simulink model "F16ASYM_Controlled"  (R2015a)
settings: Solver=ode3  SolverMode=SingleTasking  StartTime=0.0  StopTime=inf  FixedStep=T_sim  RelTol=1e-3
InitFcn:
  | load('NN_c_weights_Last_stable.mat')
StopFcn:
  | Final_results
values from neighbouring files (symbols this model uses):
  a1 = fitresult.p1    [Stall_protection.m]
  alpha_map_eval = ones(size(M_eval))*NaN    [Auto_trim_aid.m]    (also in Autotrim_maps.mat = [nan nan 0.277598136245 0.119432432992 0.0579479097061 0.027)
  beta_map_eval = ones(size(M_eval))*NaN    [Auto_trim_aid.m]    (also in Autotrim_maps.mat = [nan nan -0.00151549403324 0.00117807579006 -0.0052086799721)
  C_L_0 = fitresult.p2    [Stall_protection.m]
  G_eval = NaN*ones(size(M_sq,2),size(H_sq,2))    [Stall_protection.m]
  H_sq = unique(sort(H_sq))    [Stall_protection.m]
  H_sq_autotrim = min( F_envelope.H_1g):2000:max(F_envelope.H_1g)    [Auto_trim_aid.m]    (also in Autotrim_maps.mat = [0 2000 4000 6000 8000 10000 12000 14000 16000 18000])
  K_b_q_extrap_ACC = K_b_q_extrap    [RUN_ME.m]
  K_b_q_extrap_AoA = K_b_q_extrap    [RUN_ME.m]
  M_sq = unique(sort(M_sq))    [Stall_protection.m]
  M_sq_autotrim = 0:0.1:max(F_envelope.M_1g)    [Auto_trim_aid.m]    (also in Autotrim_maps.mat = [0 0.1 0.2 0.3 0.4 0.5 0.6 0.7 0.8 0.9 1 1.1 ... (21 element)
  T_sim = 0.02    [RUN_ME.m]
  tau_q_extrap_ACC = tau_q_extrap    [RUN_ME.m]
  tau_q_extrap_AoA = tau_q_extrap    [RUN_ME.m]
  velocity = M_eval(I,J)*a    [Auto_trim_aid.m]
undefined symbols (not defined in the file or in its folder): ACCEL, B, Earth, fi_flag_Simulink, GYRO, H_sq_sche, k_B, K_b_ACC_extrap, K_b_AoA_extrap, latitude, longitude, m, m_B, M_sq_sche, Model_used_flag, rad, s, sigbuilder_block, Stall_curve, tau_ACC_extrap, tau_AoA_extrap, Theta_1_roll_last, Theta_2_roll_last, Theta_3_roll_last, trim_control, trim_state, trim_throttle, V_Comp_A_w_z_last, V_Comp_last, V_Comp_last_ONE, V_long_lastA_w_z, V_long_lastAoA, V_roll_last, V_roll_lastMOD, V_yaw_last, W_Comp_A_w_z_last, W_Comp_last, W_long_lastA_w_z, W_long_lastAoA, W_roll_last, W_roll_lastMOD, W_yaw_last, WGS84
libraries: Adaptive_FaultTolerantControl x57, dspsigops x37, F16_Actuator_Library x14, commnoisgen2 x13, simulink x11, simulink_extras x10, dsparch4 x6, aerolibatmos2 x6, aerolibtransform2 x6, aerolibfltsims x3, dspvision x3, dspsnks4 x3
(part 9 of 14)

== system F16ASYM_Controlled/Primary Controller/P con + adaptive Crossed NN + AWU+Lim + Scheduling/Physical limitation/Moments ==
  C_L : Inport
  C_M : Inport  Port=2
  C_N : Inport  Port=3
  q : Inport  Port=4
  B span : Constant  Value=9.144
  CMA : Constant  Value=3.45
  Divide : Product  Inputs=**
  Divide1 : Product  Inputs=***
  Divide2 : Product  Inputs=**
  Divide3 : Product  Inputs=***
  Divide4 : Product  Inputs=**
  S_w : Constant  Value=27.87
  S_w1 : Constant  Value=27.87
  q1 : InportShadow  Port=4
  L : Outport
  M : Outport  Port=2
  N : Outport  Port=3
  wires:
  q/1 -> Divide1/1
  S_w/1 -> Divide1/2
  B span/1 -> Divide1/3
  C_L/1 -> Divide/1
  Divide1/1 -> Divide2/1, Divide/2
  Divide/1 -> L/1  "L"
  C_N/1 -> Divide2/2
  Divide2/1 -> N/1  "N"
  q1/1 -> Divide3/1
  S_w1/1 -> Divide3/2
  CMA/1 -> Divide3/3
  C_M/1 -> Divide4/1
  Divide3/1 -> Divide4/2
  Divide4/1 -> M/1  "M"

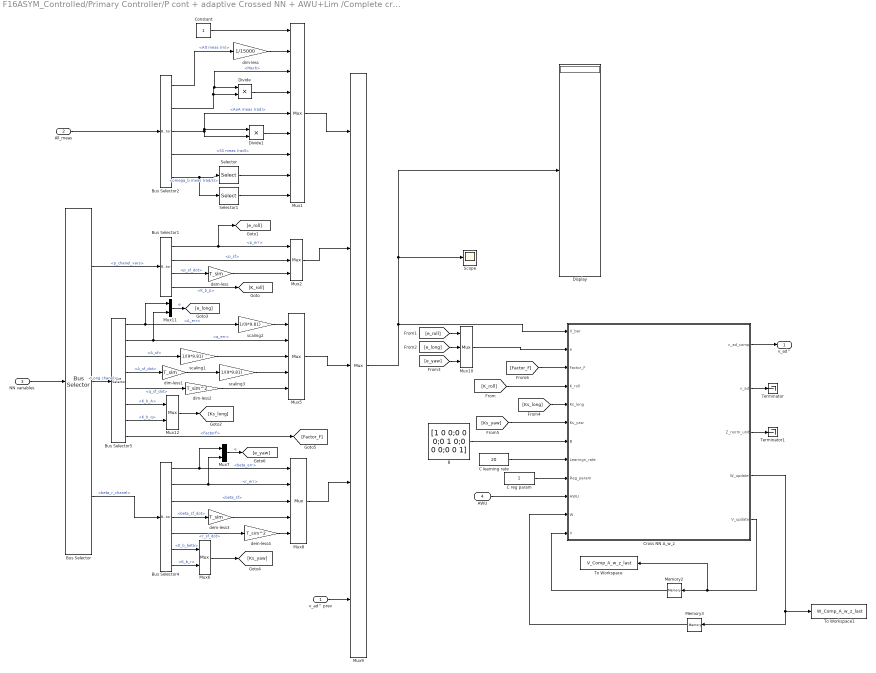
== system F16ASYM_Controlled/Primary Controller/P cont + adaptive Crossed NN + AWU+Lim /Complete crossed On-line (adaptive) multi-layer NN/Complete crossed On-line (adaptive) multi-layer NN: A_w_z ==
  v_ad^ prev : Inport
  All_meas : Inport  Port=2
  NN variables : Inport  Port=3
  AWU : Inport  Port=4
  B : Constant  Value=[1 0 0;0 0 0;0 1 0;0 0 0;0 0 1]
  Bus Selector : BusSelector  OutputSignals=p_chanel_vars,Long chanel,beta_r_chanel
  Bus Selector1 : BusSelector  OutputSignals=p_err,p_sf,p_sf_dot,K_b_p
  Bus Selector2 : BusSelector  OutputSignals=signal1.Alt meas (m),signal2.Mach,signal1.AoA meas (rad),signal1.SS meas (rad),signal1.omega_b meas (rad/s)
  Bus Selector4 : BusSelector  OutputSignals=beta_chanel vars.beta_err,r_chanel vars.r_err,beta_chanel vars.beta_sf,beta_chanel vars.beta_sf_dot,r_chanel vars.r_sf_dot,beta_chanel vars.K_b_beta,r_chanel vars.K_b_r
  Bus Selector5 : BusSelector  OutputSignals=A_chanel vars.A_err,q_chanel_vars.q_err,A_chanel vars.A_sf,A_chanel vars.A_sf_dot,q_chanel_vars.q_sf_dot,A_chanel vars.K_b_A,q_chanel_vars.K_b_q,A_chanel vars.FactorF
  C learning rate : Constant  Value=20  SampleTime=T_sim
  C reg param : Constant  SampleTime=T_sim
  Constant : Constant
  Cross NN A_w_z : MATLAB Function  TreatAsAtomicUnit=on
  Display : Display
  Divide : Product  Inputs=**
  Divide1 : Product  Inputs=**
  Memory2 : Memory  X0=V_Comp_A_w_z_last
  Memory3 : Memory  X0=W_Comp_A_w_z_last
  Mux1 : Mux  Inputs=9
  Mux10 : Mux  Inputs=3
  Mux{6..7,11..12} (4 alike) : Mux  Inputs=2
  Mux2 : Mux  Inputs=3
  Mux5 : Mux  Inputs=5
  Mux8 : Mux  Inputs=5
  Mux9 : Mux  Inputs=[9 3 5 5 3]
  Scope : Scope
      settings: SaveName=ScopeData8
  Selector : Selector  InputPortWidth=3
  Selector1 : Selector  InputPortWidth=3  Indices=3
  Terminator : Terminator
  Terminator1 : Terminator
  To Workspace : ToWorkspace  VariableName=V_Comp_A_w_z_last  SampleTime=-1
      settings: MaxDataPoints=1
  To Workspace1 : ToWorkspace  VariableName=W_Comp_A_w_z_last  SampleTime=-1
      settings: MaxDataPoints=1
  dem-less : Gain  Gain=T_sim
  dem-less3 : Gain  Gain=T_sim
  dem-less4 : Gain  Gain=T_sim^2
  dim-less : Gain  Gain=1/15000
  dim-less1 : Gain  Gain=T_sim
  dim-less2 : Gain  Gain=T_sim^2
  scaling1 : Gain  Gain=1/(9*9.81)
  scaling2 : Gain  Gain=1/(9*9.81)
  scaling3 : Gain  Gain=1/(9*9.81)
  v_ad^ : Outport
  wires:
  [Factor_F] -> Cross NN A_w_z/3(Factor_F)
  Bus Selector5/8 -> [Factor_F]  "<FactorF>"
  scaling3/1 -> Mux5/4
  dim-less2/1 -> Mux5/5
  scaling1/1 -> Mux5/3
  Mux11/1 -> [e_long]  "e"
  Bus Selector/2 -> Bus Selector5/1  "<Long chanel>"
  Bus Selector5/1 -> Mux11/1, scaling2/1  "<A_err>"
  Bus Selector5/2 -> Mux11/2, Mux5/2  "<q_err>"
  Bus Selector5/3 -> scaling1/1  "<A_sf>"
  Bus Selector5/4 -> dim-less1/1  "<A_sf_dot>"
  Bus Selector5/5 -> dim-less2/1  "<q_sf_dot>"
  Bus Selector5/7 -> Mux12/2  "<K_b_q>"
  Bus Selector5/6 -> Mux12/1  "<K_b_A>"
  scaling2/1 -> Mux5/1
  dim-less1/1 -> scaling3/1
  Selector1/1 -> Mux1/9
  [Ks_yaw] -> Cross NN A_w_z/6(Ks_yaw)
  [Ks_long] -> Cross NN A_w_z/5(Ks_long)
  [K_roll] -> Cross NN A_w_z/4(K_roll)
  [e_yaw] -> Mux10/3
  [e_long] -> Mux10/2
  [e_roll] -> Mux10/1
  Mux10/1 -> Cross NN A_w_z/2(e)
  Cross NN A_w_z/4(W_update) -> To Workspace1/1, Memory3/1
  Cross NN A_w_z/5(V_update) -> Memory2/1, To Workspace/1
  Cross NN A_w_z/2(v_ad) -> Terminator/1
  B/1 -> Cross NN A_w_z/7(B)
  Memory3/1 -> Cross NN A_w_z/11(W)
  Memory2/1 -> Cross NN A_w_z/12(V)
  Cross NN A_w_z/1(v_ad_comp) -> v_ad^/1
  C learning rate/1 -> Cross NN A_w_z/8(Learnign_rate)
  C reg param/1 -> Cross NN A_w_z/9(Reg_param)
  Cross NN A_w_z/3(Z_norm_unit) -> Terminator1/1
  Mux9/1 -> Cross NN A_w_z/1(X_bar), Display/1, Scope/1
  v_ad^ prev/1 -> Mux9/5
  Mux8/1 -> Mux9/4
  Mux5/1 -> Mux9/3
  Mux2/1 -> Mux9/2
  Mux1/1 -> Mux9/1
  dem-less4/1 -> Mux8/5
  Mux7/1 -> [e_yaw]  "e"
  Bus Selector4/2 -> Mux7/2, Mux8/2  "<r_err>"
  Bus Selector4/1 -> Mux7/1, Mux8/1  "<beta_err>"
  Mux6/1 -> [Ks_yaw]
  Bus Selector4/6 -> Mux6/1  "<K_b_beta>"
  Bus Selector4/7 -> Mux6/2  "<K_b_r>"
  Bus Selector4/5 -> dem-less4/1  "<r_sf_dot>"
  Bus Selector4/4 -> dem-less3/1  "<beta_sf_dot>"
  Bus Selector4/3 -> Mux8/3  "<beta_sf>"
  dem-less3/1 -> Mux8/4
  Mux12/1 -> [Ks_long]
  dem-less/1 -> Mux2/3
  Bus Selector1/1 -> Mux2/1, [e_roll]  "<p_err>"
  Bus Selector1/2 -> Mux2/2  "<p_sf>"
  Bus Selector1/4 -> [K_roll]  "<K_b_p>"
  Bus Selector2/3 -> Divide1/2, Mux1/5, Divide1/1  "<AoA meas (rad)>"
  Bus Selector2/2 -> Divide/1, Mux1/3, Divide/2  "<Mach>"
  Bus Selector2/4 -> Mux1/7  "<SS meas (rad)>"
  Selector/1 -> Mux1/8
  Bus Selector1/3 -> dem-less/1  "<p_sf_dot>"
  Constant/1 -> Mux1/1
  All_meas/1 -> Bus Selector2/1
  Bus Selector2/1 -> dim-less/1  "<Alt meas (m)>"
  Divide/1 -> Mux1/4
  Divide1/1 -> Mux1/6
  dim-less/1 -> Mux1/2
  Bus Selector2/5 -> Selector/1, Selector1/1  "<omega_b meas (rad/s)>"
  NN variables/1 -> Bus Selector/1
  Bus Selector/1 -> Bus Selector1/1  "<p_chanel_vars>"
  Bus Selector/3 -> Bus Selector4/1  "<beta_r_chanel>"
  AWU/1 -> Cross NN A_w_z/10(AWU)

== system F16ASYM_Controlled/Primary Controller/P cont + adaptive Crossed NN + AWU+Lim /Complete crossed On-line (adaptive) multi-layer NN/Complete crossed On-line (adaptive) multi-layer NN: AoA ==
  v_ad^ prev : Inport
  All_meas : Inport  Port=2
  NN variables : Inport  Port=3
  AWU : Inport  Port=4
  B : Constant  Value=[1 0 0;0 0 0;0 1 0;0 0 0;0 0 1]
  Bus Selector : BusSelector  OutputSignals=p_chanel_vars,Long chanel,beta_r_chanel
  Bus Selector1 : BusSelector  OutputSignals=p_err,p_sf,p_sf_dot,K_b_p
  Bus Selector2 : BusSelector  OutputSignals=signal1.Alt meas (m),signal2.Mach,signal1.AoA meas (rad),signal1.SS meas (rad),signal1.omega_b meas (rad/s)
  Bus Selector3 : BusSelector  OutputSignals=alpha_chanel vars.alpha_err,q_chanel_vars.q_err,alpha_chanel vars.alpha_sf,alpha_chanel vars.alpha_sf_dot,q_chanel_vars.q_sf_dot,alpha_chanel vars.K_b_alpha,q_chanel_vars.K_b_q
  Bus Selector4 : BusSelector  OutputSignals=beta_chanel vars.beta_err,r_chanel vars.r_err,beta_chanel vars.beta_sf,beta_chanel vars.beta_sf_dot,r_chanel vars.r_sf_dot,beta_chanel vars.K_b_beta,r_chanel vars.K_b_r
  C Learning rate : Constant  Value=30  SampleTime=T_sim
  C Reg param : Constant  SampleTime=T_sim
  Constant : Constant
  Cross NN : MATLAB Function  TreatAsAtomicUnit=on
  Display : Display
  Divide : Product  Inputs=**
  Divide1 : Product  Inputs=**
  Memory2 : Memory  X0=V_Comp_last
  Memory3 : Memory  X0=W_Comp_last
  Mux1 : Mux  Inputs=9
  Mux10 : Mux  Inputs=3
  Mux2 : Mux  Inputs=3
  Mux{3..4,6..7} (4 alike) : Mux  Inputs=2
  Mux5 : Mux  Inputs=5
  Mux8 : Mux  Inputs=5
  Mux9 : Mux  Inputs=[9 3 5 5 3]
  Scope : Scope
      settings: SaveName=ScopeData8
  Selector : Selector  InputPortWidth=3
  Selector1 : Selector  InputPortWidth=3  Indices=3
  Terminator : Terminator
  Terminator1 : Terminator
  To Workspace : ToWorkspace  VariableName=V_Comp_last  SampleTime=-1
      settings: MaxDataPoints=1
  To Workspace1 : ToWorkspace  VariableName=W_Comp_last  SampleTime=-1
      settings: MaxDataPoints=1
  To Workspace2 : ToWorkspace  VariableName=W_online  SaveFormat=Timeseries  SampleTime=-1
  To Workspace3 : ToWorkspace  VariableName=V_online  SaveFormat=Timeseries  SampleTime=-1
  dem-less : Gain  Gain=T_sim
  dem-less1 : Gain  Gain=T_sim
  dem-less2 : Gain  Gain=T_sim^2
  dem-less3 : Gain  Gain=T_sim
  dem-less4 : Gain  Gain=T_sim^2
  dim-less : Gain  Gain=1/15000
  v_ad^ : Outport
  wires:
  Bus Selector/3 -> Bus Selector4/1  "<beta_r_chanel>"
  Bus Selector/2 -> Bus Selector3/1  "<Long chanel>"
  Bus Selector/1 -> Bus Selector1/1  "<p_chanel_vars>"
  NN variables/1 -> Bus Selector/1
  Bus Selector2/5 -> Selector1/1, Selector/1  "<omega_b meas (rad/s)>"
  dim-less/1 -> Mux1/2
  Divide1/1 -> Mux1/6
  Divide/1 -> Mux1/4
  Bus Selector2/1 -> dim-less/1  "<Alt meas (m)>"
  All_meas/1 -> Bus Selector2/1
  Constant/1 -> Mux1/1
  Bus Selector1/3 -> dem-less/1  "<p_sf_dot>"
  Selector/1 -> Mux1/8
  Bus Selector2/4 -> Mux1/7  "<SS meas (rad)>"
  Bus Selector2/2 -> Divide/2, Mux1/3, Divide/1  "<Mach>"
  Bus Selector2/3 -> Divide1/1, Mux1/5, Divide1/2  "<AoA meas (rad)>"
  Bus Selector1/4 -> [K_roll]  "<K_b_p>"
  Bus Selector1/2 -> Mux2/2  "<p_sf>"
  Bus Selector1/1 -> [e_roll], Mux2/1  "<p_err>"
  dem-less/1 -> Mux2/3
  dem-less2/1 -> Mux5/5
  dem-less1/1 -> Mux5/4
  Mux4/1 -> [Ks_long]
  Bus Selector3/6 -> Mux4/1  "<K_b_alpha>"
  Bus Selector3/7 -> Mux4/2  "<K_b_q>"
  Bus Selector3/5 -> dem-less2/1  "<q_sf_dot>"
  Bus Selector3/4 -> dem-less1/1  "<alpha_sf_dot>"
  Bus Selector3/1 -> Mux5/1, Mux3/1  "<alpha_err>"
  Bus Selector3/2 -> Mux5/2, Mux3/2  "<q_err>"
  Bus Selector3/3 -> Mux5/3  "<alpha_sf>"
  Mux3/1 -> [e_long]  "e"
  dem-less3/1 -> Mux8/4
  Bus Selector4/3 -> Mux8/3  "<beta_sf>"
  Bus Selector4/4 -> dem-less3/1  "<beta_sf_dot>"
  Bus Selector4/5 -> dem-less4/1  "<r_sf_dot>"
  Bus Selector4/7 -> Mux6/2  "<K_b_r>"
  Bus Selector4/6 -> Mux6/1  "<K_b_beta>"
  Mux6/1 -> [Ks_yaw]
  Bus Selector4/1 -> Mux8/1, Mux7/1  "<beta_err>"
  Bus Selector4/2 -> Mux8/2, Mux7/2  "<r_err>"
  Mux7/1 -> [e_yaw]  "e"
  dem-less4/1 -> Mux8/5
  Mux1/1 -> Mux9/1
  Mux2/1 -> Mux9/2
  Mux5/1 -> Mux9/3
  Mux8/1 -> Mux9/4
  v_ad^ prev/1 -> Mux9/5
  Mux9/1 -> Scope/1, Display/1, Cross NN/1(X_bar)
  Cross NN/3(Z_norm_unit) -> Terminator1/1
  C Reg param/1 -> Cross NN/8(Reg_param)
  C Learning rate/1 -> Cross NN/7(Learnign_rate)
  Cross NN/1(v_ad_comp) -> v_ad^/1
  Memory2/1 -> Cross NN/11(V)
  Memory3/1 -> Cross NN/10(W)
  B/1 -> Cross NN/6(B)
  Cross NN/2(v_ad) -> Terminator/1
  Cross NN/5(V_update) -> To Workspace3/1, To Workspace/1, Memory2/1
  Cross NN/4(W_update) -> To Workspace2/1, Memory3/1, To Workspace1/1
  Mux10/1 -> Cross NN/2(e)
  [e_roll] -> Mux10/1
  [e_long] -> Mux10/2
  [e_yaw] -> Mux10/3
  [K_roll] -> Cross NN/3(K_roll)
  [Ks_long] -> Cross NN/4(Ks_long)
  [Ks_yaw] -> Cross NN/5(Ks_yaw)
  Selector1/1 -> Mux1/9
  AWU/1 -> Cross NN/9(AWU)

== system F16ASYM_Controlled/Primary Controller/P cont + adaptive Crossed NN + AWU+Lim /Long Dyn Inversion: alpha_dot ->q/Completed ==
  alpha_dot_c : Inport
  All_meas : Inport  Port=2
  A_w_z : Selector  InputPortWidth=3  Indices=3
  Add : Sum
  Bus Selector : BusSelector  OutputSignals=signal1.AoA meas (rad),signal1.omega_b meas (rad/s),signal1.SS meas (rad),signal1.V_TAS (m/s),signal2.A_w_CG
  Display : Display
  Display1 : Display
  Display2 : Display
  Divide{,1..3} (4 alike) : Product  Inputs=**
  Divide4 : Product  Inputs=/*
  Selector : Selector  InputPortWidth=3
  Selector1 : Selector  InputPortWidth=3  Indices=3
  Trigonometric Function : Trigonometry  Operator=sincos
  Trigonometric Function1 : Trigonometry  Operator=tan
  Trigonometric Function2 : Trigonometry  Operator=cos
  "q_c " : Sum  Inputs=++-
  q_c : Outport
  wires:
  Trigonometric Function/1 -> Divide1/1
  Bus Selector/1 -> Trigonometric Function/1  "<AoA meas (rad)>"
  Selector/1 -> Divide/2
  Bus Selector/2 -> Selector1/1, Selector/1  "<omega_b meas (rad/s)>"
  Divide2/1 -> "q_c "/2, Display1/1
  Selector1/1 -> Divide1/2
  Divide3/1 -> Divide4/1
  alpha_dot_c/1 -> "q_c "/1, Display/1
  All_meas/1 -> Bus Selector/1
  Bus Selector/5 -> A_w_z/1  "<A_w_CG>"
  Bus Selector/3 -> Trigonometric Function1/1, Trigonometric Function2/1  "<SS meas (rad)>"
  Divide4/1 -> "q_c "/3
  "q_c "/1 -> q_c/1
  Divide/1 -> Add/1
  Bus Selector/4 -> Divide3/2  "<V_TAS (m/s)>"
  Add/1 -> Divide2/1
  Trigonometric Function1/1 -> Divide2/2
  Divide1/1 -> Add/2
  Trigonometric Function2/1 -> Divide3/1
  Trigonometric Function/2 -> Divide/1
  A_w_z/1 -> Display2/1, Divide4/2

== system F16ASYM_Controlled/Primary Controller/P cont + adaptive Crossed NN + AWU+Lim /Long Dyn Inversion: alpha_dot ->q/Simplified ==
  alpha_dot_c : Inport
  All_meas : Inport  Port=2
  A_b_z : Selector  InputPortWidth=3  Indices=3
  Bus Selector : BusSelector  OutputSignals=signal2.A_b_CG,signal1.V_TAS (m/s)
  Display : Display
  Divide4 : Product  Inputs=*/
  "q_c " : Sum  Inputs=+-
  q_c : Outport
  wires:
  "q_c "/1 -> q_c/1
  All_meas/1 -> Bus Selector/1
  alpha_dot_c/1 -> "q_c "/1, Display/1
  Bus Selector/2 -> Divide4/2  "<V_TAS (m/s)>"
  Divide4/1 -> "q_c "/2
  A_b_z/1 -> Divide4/1  "A_b_z"
  Bus Selector/1 -> A_b_z/1  "<A_b_CG>"

== system F16ASYM_Controlled/Primary Controller/P cont + adaptive Crossed NN + AWU+Lim /Longitudinal Controller: AoA or A_w_z/Longitudinal controller in A_w_z ==
  A_w_z des : Inport
  AoA des (rad) : Inport  Port=2
  Anti-windup A_w_z : Inport  Port=3
  Anti-windup AoA : Inport  Port=4
  All meas : Inport  Port=5
  Accel rate --> AoA rate! : Subsystem
  Bus Creator : BusCreator  Inputs=5
  Bus Selector : BusSelector  OutputSignals=signal2.A_w_CG
  Divide : Product  Inputs=**
  Gain : Gain  Gain=-1
  Ground : Ground
  Ref Model and P Controller : Adaptive_FaultTolerantControl/Ref Model and P Controller  tau=2  y_i=0  K_f=1  K_b=1
  Selector : Selector  InputPortWidth=3  Indices=3
  Stall protection : Subsystem  Commented=on
  Sum : Sum  Inputs=+-|
  Terminator : Terminator
  Terminator1 : Terminator
  Terminator2 : Terminator
  A_chanel vars : Outport
  alpha_chanel vars : Outport  Port=2
  alpha_dot_c : Outport  Port=3
  wires:
  Anti-windup AoA/1 -> Terminator1/1
  AoA des (rad)/1 -> Terminator/1
  Selector/1 -> Gain/1
  Gain/1 -> Ref Model and P Controller/2
  Bus Selector/1 -> Selector/1  "<A_w_CG>"
  Anti-windup A_w_z/1 -> Terminator2/1
  A_w_z des/1 -> Ref Model and P Controller/1
  Ref Model and P Controller/1 -> Divide/1
  Ref Model and P Controller/2 -> Bus Creator/1  "A_sf_dot"
  Ref Model and P Controller/3 -> Bus Creator/2, Sum/1  "A_sf"
  Sum/1 -> Bus Creator/3  "A_err"
  Ref Model and P Controller/4 -> Sum/2
  Ref Model and P Controller/5 -> Bus Creator/4  "K_b_A"
  Bus Creator/1 -> A_chanel vars/1
  Ground/1 -> alpha_chanel vars/1
  Divide/1 -> alpha_dot_c/1
  Accel rate --> AoA rate!/1(A_w  to AoA rates factor) -> Bus Creator/5, Divide/2  "FactorF"
  All meas/1 -> Bus Selector/1, Stall protection/2(All meas), Accel rate --> AoA rate!/1(All_meas)

== system F16ASYM_Controlled/Primary Controller/P cont + adaptive Crossed NN + AWU+Lim /Longitudinal Controller: AoA or A_w_z/Longitudinal controller in AoA ==
  A_w_z des : Inport
  AoA des (rad) : Inport  Port=2
  Anti-windup A_w_z : Inport  Port=3
  Anti-windup AoA : Inport  Port=4
  All meas : Inport  Port=5
  Bus Creator : BusCreator
  Bus Selector : BusSelector  OutputSignals=signal1.AoA meas (rad)
  Ground : Ground
  Ref Model and P Controller : Adaptive_FaultTolerantControl/Ref Model and P Controller  tau=0.6  y_i=trim_state(8)  K_f=1  K_b=3.5
  Sum : Sum  Inputs=+-|
  Terminator : Terminator
  Terminator1 : Terminator
  Terminator2 : Terminator
  A_chanel vars : Outport
  alpha_chanel vars : Outport  Port=2
  alpha_dot_c : Outport  Port=3
  wires:
  All meas/1 -> Bus Selector/1
  Ref Model and P Controller/1 -> alpha_dot_c/1
  Bus Selector/1 -> Ref Model and P Controller/2  "<AoA meas (rad)>"
  AoA des (rad)/1 -> Ref Model and P Controller/1
  A_w_z des/1 -> Terminator/1
  Anti-windup A_w_z/1 -> Terminator1/1
  Anti-windup AoA/1 -> Terminator2/1
  Ref Model and P Controller/2 -> Bus Creator/1  "alpha_sf_dot"
  Ref Model and P Controller/3 -> Sum/1, Bus Creator/2  "alpha_sf"
  Sum/1 -> Bus Creator/3  "alpha_err"
  Bus Creator/1 -> alpha_chanel vars/1
  Ref Model and P Controller/4 -> Sum/2
  Ref Model and P Controller/5 -> Bus Creator/4  "K_b_alpha"
  Ground/1 -> A_chanel vars/1

== system F16ASYM_Controlled/Primary Controller/P cont + adaptive Crossed NN + AWU+Lim /Physical limitation/Moments ==
  C_L : Inport
  C_M : Inport  Port=2
  C_N : Inport  Port=3
  q : Inport  Port=4
  B span : Constant  Value=9.144
  CMA : Constant  Value=3.45
  Divide : Product  Inputs=**
  Divide1 : Product  Inputs=***
  Divide2 : Product  Inputs=**
  Divide3 : Product  Inputs=***
  Divide4 : Product  Inputs=**
  S_w : Constant  Value=27.87
  S_w1 : Constant  Value=27.87
  q1 : InportShadow  Port=4
  L : Outport
  M : Outport  Port=2
  N : Outport  Port=3
  wires:
  Divide4/1 -> M/1  "M"
  Divide3/1 -> Divide4/2
  C_M/1 -> Divide4/1
  CMA/1 -> Divide3/3
  S_w1/1 -> Divide3/2
  q1/1 -> Divide3/1
  Divide2/1 -> N/1  "N"
  C_N/1 -> Divide2/2
  Divide/1 -> L/1  "L"
  Divide1/1 -> Divide/2, Divide2/1
  C_L/1 -> Divide/1
  B span/1 -> Divide1/3
  S_w/1 -> Divide1/2
  q/1 -> Divide1/1

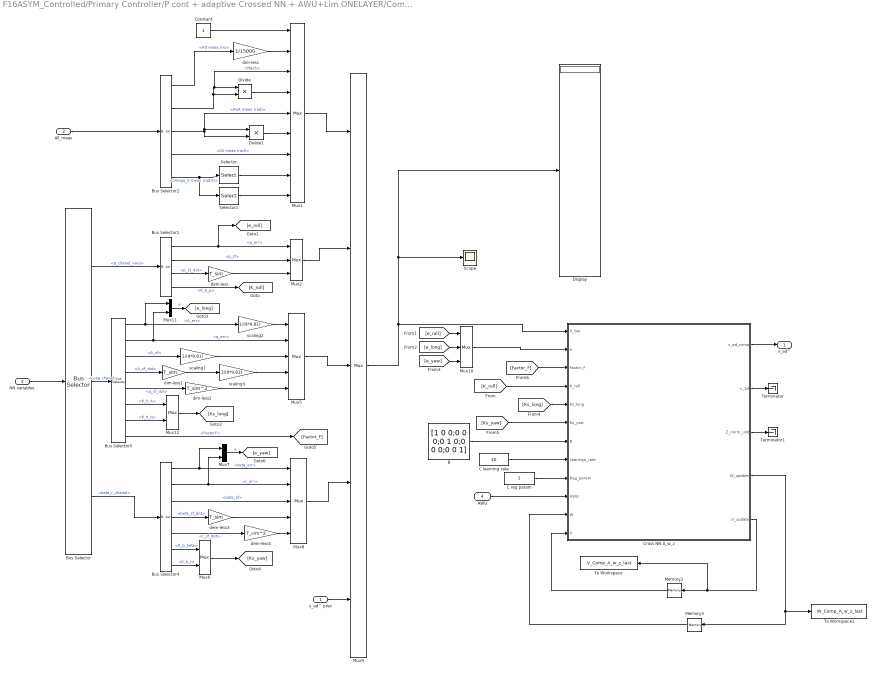
== system F16ASYM_Controlled/Primary Controller/P cont + adaptive Crossed NN + AWU+Lim ONELAYER/Complete crossed On-line (adaptive) multi-layer NN/Complete crossed On-line (adaptive) multi-layer NN: A_w_z ==
  v_ad^ prev : Inport
  All_meas : Inport  Port=2
  NN variables : Inport  Port=3
  AWU : Inport  Port=4
  B : Constant  Value=[1 0 0;0 0 0;0 1 0;0 0 0;0 0 1]
  Bus Selector : BusSelector  OutputSignals=p_chanel_vars,Long chanel,beta_r_chanel
  Bus Selector1 : BusSelector  OutputSignals=p_err,p_sf,p_sf_dot,K_b_p
  Bus Selector2 : BusSelector  OutputSignals=signal1.Alt meas (m),signal2.Mach,signal1.AoA meas (rad),signal1.SS meas (rad),signal1.omega_b meas (rad/s)
  Bus Selector4 : BusSelector  OutputSignals=beta_chanel vars.beta_err,r_chanel vars.r_err,beta_chanel vars.beta_sf,beta_chanel vars.beta_sf_dot,r_chanel vars.r_sf_dot,beta_chanel vars.K_b_beta,r_chanel vars.K_b_r
  Bus Selector5 : BusSelector  OutputSignals=A_chanel vars.A_err,q_chanel_vars.q_err,A_chanel vars.A_sf,A_chanel vars.A_sf_dot,q_chanel_vars.q_sf_dot,A_chanel vars.K_b_A,q_chanel_vars.K_b_q,A_chanel vars.FactorF
  C learning rate : Constant  Value=20  SampleTime=T_sim
  C reg param : Constant  SampleTime=T_sim
  Constant : Constant
  Cross NN A_w_z : MATLAB Function  TreatAsAtomicUnit=on
  Display : Display
  Divide : Product  Inputs=**
  Divide1 : Product  Inputs=**
  Memory2 : Memory  X0=V_Comp_A_w_z_last
  Memory3 : Memory  X0=W_Comp_A_w_z_last
  Mux1 : Mux  Inputs=9
  Mux10 : Mux  Inputs=3
  Mux{6..7,11..12} (4 alike) : Mux  Inputs=2
  Mux2 : Mux  Inputs=3
  Mux5 : Mux  Inputs=5
  Mux8 : Mux  Inputs=5
  Mux9 : Mux  Inputs=[9 3 5 5 3]
  Scope : Scope
      settings: SaveName=ScopeData8
  Selector : Selector  InputPortWidth=3
  Selector1 : Selector  InputPortWidth=3  Indices=3
  Terminator : Terminator
  Terminator1 : Terminator
  To Workspace : ToWorkspace  VariableName=V_Comp_A_w_z_last  SampleTime=-1
      settings: MaxDataPoints=1
  To Workspace1 : ToWorkspace  VariableName=W_Comp_A_w_z_last  SampleTime=-1
      settings: MaxDataPoints=1
  dem-less : Gain  Gain=T_sim
  dem-less3 : Gain  Gain=T_sim
  dem-less4 : Gain  Gain=T_sim^2
  dim-less : Gain  Gain=1/15000
  dim-less1 : Gain  Gain=T_sim
  dim-less2 : Gain  Gain=T_sim^2
  scaling1 : Gain  Gain=1/(9*9.81)
  scaling2 : Gain  Gain=1/(9*9.81)
  scaling3 : Gain  Gain=1/(9*9.81)
  v_ad^ : Outport
  wires:
  [Factor_F] -> Cross NN A_w_z/3(Factor_F)
  Bus Selector5/8 -> [Factor_F]  "<FactorF>"
  scaling3/1 -> Mux5/4
  dim-less2/1 -> Mux5/5
  scaling1/1 -> Mux5/3
  Mux11/1 -> [e_long]  "e"
  Bus Selector/2 -> Bus Selector5/1  "<Long chanel>"
  Bus Selector5/1 -> Mux11/1, scaling2/1  "<A_err>"
  Bus Selector5/2 -> Mux11/2, Mux5/2  "<q_err>"
  Bus Selector5/3 -> scaling1/1  "<A_sf>"
  Bus Selector5/4 -> dim-less1/1  "<A_sf_dot>"
  Bus Selector5/5 -> dim-less2/1  "<q_sf_dot>"
  Bus Selector5/7 -> Mux12/2  "<K_b_q>"
  Bus Selector5/6 -> Mux12/1  "<K_b_A>"
  scaling2/1 -> Mux5/1
  dim-less1/1 -> scaling3/1
  Selector1/1 -> Mux1/9
  [Ks_yaw] -> Cross NN A_w_z/6(Ks_yaw)
  [Ks_long] -> Cross NN A_w_z/5(Ks_long)
  [K_roll] -> Cross NN A_w_z/4(K_roll)
  [e_yaw] -> Mux10/3
  [e_long] -> Mux10/2
  [e_roll] -> Mux10/1
  Mux10/1 -> Cross NN A_w_z/2(e)
  Cross NN A_w_z/4(W_update) -> To Workspace1/1, Memory3/1
  Cross NN A_w_z/5(V_update) -> Memory2/1, To Workspace/1
  Cross NN A_w_z/2(v_ad) -> Terminator/1
  B/1 -> Cross NN A_w_z/7(B)
  Memory3/1 -> Cross NN A_w_z/11(W)
  Memory2/1 -> Cross NN A_w_z/12(V)
  Cross NN A_w_z/1(v_ad_comp) -> v_ad^/1
  C learning rate/1 -> Cross NN A_w_z/8(Learnign_rate)
  C reg param/1 -> Cross NN A_w_z/9(Reg_param)
  Cross NN A_w_z/3(Z_norm_unit) -> Terminator1/1
  Mux9/1 -> Cross NN A_w_z/1(X_bar), Display/1, Scope/1
  v_ad^ prev/1 -> Mux9/5
  Mux8/1 -> Mux9/4
  Mux5/1 -> Mux9/3
  Mux2/1 -> Mux9/2
  Mux1/1 -> Mux9/1
  dem-less4/1 -> Mux8/5
  Mux7/1 -> [e_yaw]  "e"
  Bus Selector4/2 -> Mux7/2, Mux8/2  "<r_err>"
  Bus Selector4/1 -> Mux7/1, Mux8/1  "<beta_err>"
  Mux6/1 -> [Ks_yaw]
  Bus Selector4/6 -> Mux6/1  "<K_b_beta>"
  Bus Selector4/7 -> Mux6/2  "<K_b_r>"
  Bus Selector4/5 -> dem-less4/1  "<r_sf_dot>"
  Bus Selector4/4 -> dem-less3/1  "<beta_sf_dot>"
  Bus Selector4/3 -> Mux8/3  "<beta_sf>"
  dem-less3/1 -> Mux8/4
  Mux12/1 -> [Ks_long]
  dem-less/1 -> Mux2/3
  Bus Selector1/1 -> Mux2/1, [e_roll]  "<p_err>"
  Bus Selector1/2 -> Mux2/2  "<p_sf>"
  Bus Selector1/4 -> [K_roll]  "<K_b_p>"
  Bus Selector2/3 -> Divide1/2, Mux1/5, Divide1/1  "<AoA meas (rad)>"
  Bus Selector2/2 -> Divide/1, Mux1/3, Divide/2  "<Mach>"
  Bus Selector2/4 -> Mux1/7  "<SS meas (rad)>"
  Selector/1 -> Mux1/8
  Bus Selector1/3 -> dem-less/1  "<p_sf_dot>"
  Constant/1 -> Mux1/1
  All_meas/1 -> Bus Selector2/1
  Bus Selector2/1 -> dim-less/1  "<Alt meas (m)>"
  Divide/1 -> Mux1/4
  Divide1/1 -> Mux1/6
  dim-less/1 -> Mux1/2
  Bus Selector2/5 -> Selector/1, Selector1/1  "<omega_b meas (rad/s)>"
  NN variables/1 -> Bus Selector/1
  Bus Selector/1 -> Bus Selector1/1  "<p_chanel_vars>"
  Bus Selector/3 -> Bus Selector4/1  "<beta_r_chanel>"
  AWU/1 -> Cross NN A_w_z/10(AWU)

== system F16ASYM_Controlled/Primary Controller/P cont + adaptive Crossed NN + AWU+Lim ONELAYER/Complete crossed On-line (adaptive) multi-layer NN/Complete crossed On-line (adaptive) multi-layer NN: AoA ==
  v_ad^ prev : Inport
  All_meas : Inport  Port=2
  NN variables : Inport  Port=3
  AWU : Inport  Port=4
  B : Constant  Value=[1 0 0;0 0 0;0 1 0;0 0 0;0 0 1]
  Bus Selector : BusSelector  OutputSignals=p_chanel_vars,Long chanel,beta_r_chanel
  Bus Selector1 : BusSelector  OutputSignals=p_err,p_sf,p_sf_dot,K_b_p
  Bus Selector2 : BusSelector  OutputSignals=signal1.Alt meas (m),signal2.Mach,signal1.AoA meas (rad),signal1.SS meas (rad),signal1.omega_b meas (rad/s)
  Bus Selector3 : BusSelector  OutputSignals=alpha_chanel vars.alpha_err,q_chanel_vars.q_err,alpha_chanel vars.alpha_sf,alpha_chanel vars.alpha_sf_dot,q_chanel_vars.q_sf_dot,alpha_chanel vars.K_b_alpha,q_chanel_vars.K_b_q
  Bus Selector4 : BusSelector  OutputSignals=beta_chanel vars.beta_err,r_chanel vars.r_err,beta_chanel vars.beta_sf,beta_chanel vars.beta_sf_dot,r_chanel vars.r_sf_dot,beta_chanel vars.K_b_beta,r_chanel vars.K_b_r
  C Learning rate : Constant  Value=30  SampleTime=T_sim
  C Reg param : Constant  SampleTime=T_sim
  Constant : Constant
  Cross NN : MATLAB Function  TreatAsAtomicUnit=on
  Display : Display
  Divide : Product  Inputs=**
  Divide1 : Product  Inputs=**
  Memory2 : Memory  X0=V_Comp_last_ONE
  Mux1 : Mux  Inputs=9
  Mux10 : Mux  Inputs=3
  Mux2 : Mux  Inputs=3
  Mux{3..4,6..7} (4 alike) : Mux  Inputs=2
  Mux5 : Mux  Inputs=5
  Mux8 : Mux  Inputs=5
  Mux9 : Mux  Inputs=[9 3 5 5 3]
  Scope : Scope
      settings: SaveName=ScopeData8
  Selector : Selector  InputPortWidth=3
  Selector1 : Selector  InputPortWidth=3  Indices=3
  Terminator2 : Terminator
  To Workspace : ToWorkspace  VariableName=V_Comp_last_ONE  SampleTime=-1
      settings: MaxDataPoints=1
  dem-less : Gain  Gain=T_sim
  dem-less1 : Gain  Gain=T_sim
  dem-less2 : Gain  Gain=T_sim^2
  dem-less3 : Gain  Gain=T_sim
  dem-less4 : Gain  Gain=T_sim^2
  dim-less : Gain  Gain=1/15000
  v_ad^ : Outport
  wires:
  Bus Selector/3 -> Bus Selector4/1  "<beta_r_chanel>"
  Bus Selector/2 -> Bus Selector3/1  "<Long chanel>"
  Bus Selector/1 -> Bus Selector1/1  "<p_chanel_vars>"
  NN variables/1 -> Bus Selector/1
  Bus Selector2/5 -> Selector1/1, Selector/1  "<omega_b meas (rad/s)>"
  dim-less/1 -> Mux1/2
  Divide1/1 -> Mux1/6
  Divide/1 -> Mux1/4
  Bus Selector2/1 -> dim-less/1  "<Alt meas (m)>"
  All_meas/1 -> Bus Selector2/1
  Constant/1 -> Mux1/1
  Bus Selector1/3 -> dem-less/1  "<p_sf_dot>"
  Selector/1 -> Mux1/8
  Bus Selector2/4 -> Mux1/7  "<SS meas (rad)>"
  Bus Selector2/2 -> Divide/2, Mux1/3, Divide/1  "<Mach>"
  Bus Selector2/3 -> Divide1/1, Mux1/5, Divide1/2  "<AoA meas (rad)>"
  Bus Selector1/4 -> [K_roll]  "<K_b_p>"
  Bus Selector1/2 -> Mux2/2  "<p_sf>"
  Bus Selector1/1 -> [e_roll], Mux2/1  "<p_err>"
  dem-less/1 -> Mux2/3
  dem-less2/1 -> Mux5/5
  dem-less1/1 -> Mux5/4
  Mux4/1 -> [Ks_long]
  Bus Selector3/6 -> Mux4/1  "<K_b_alpha>"
  Bus Selector3/7 -> Mux4/2  "<K_b_q>"
  Bus Selector3/5 -> dem-less2/1  "<q_sf_dot>"
  Bus Selector3/4 -> dem-less1/1  "<alpha_sf_dot>"
  Bus Selector3/1 -> Mux5/1, Mux3/1  "<alpha_err>"
  Bus Selector3/2 -> Mux5/2, Mux3/2  "<q_err>"
  Bus Selector3/3 -> Mux5/3  "<alpha_sf>"
  Mux3/1 -> [e_long]  "e"
  dem-less3/1 -> Mux8/4
  Bus Selector4/3 -> Mux8/3  "<beta_sf>"
  Bus Selector4/4 -> dem-less3/1  "<beta_sf_dot>"
  Bus Selector4/5 -> dem-less4/1  "<r_sf_dot>"
  Bus Selector4/7 -> Mux6/2  "<K_b_r>"
  Bus Selector4/6 -> Mux6/1  "<K_b_beta>"
  Mux6/1 -> [Ks_yaw]
  Bus Selector4/1 -> Mux8/1, Mux7/1  "<beta_err>"
  Bus Selector4/2 -> Mux8/2, Mux7/2  "<r_err>"
  Mux7/1 -> [e_yaw]  "e"
  dem-less4/1 -> Mux8/5
  Mux1/1 -> Mux9/1
  Mux2/1 -> Mux9/2
  Mux5/1 -> Mux9/3
  Mux8/1 -> Mux9/4
  v_ad^ prev/1 -> Mux9/5
  Mux9/1 -> Scope/1, Display/1, Cross NN/1(X_bar)
  C Reg param/1 -> Cross NN/8(Reg_param)
  C Learning rate/1 -> Cross NN/7(Learnign_rate)
  Memory2/1 -> Cross NN/10(V)
  B/1 -> Cross NN/6(B)
  Cross NN/2(v_ad) -> v_ad^/1
  Cross NN/3(V_update) -> To Workspace/1, Memory2/1
  Mux10/1 -> Cross NN/2(e)
  [e_roll] -> Mux10/1
  [e_long] -> Mux10/2
  [e_yaw] -> Mux10/3
  [K_roll] -> Cross NN/3(K_roll)
  [Ks_long] -> Cross NN/4(Ks_long)
  [Ks_yaw] -> Cross NN/5(Ks_yaw)
  Selector1/1 -> Mux1/9
  AWU/1 -> Cross NN/9(AWU)
  Cross NN/1(v_ad_comp) -> Terminator2/1

== system F16ASYM_Controlled/Primary Controller/P cont + adaptive Crossed NN + AWU+Lim ONELAYER/Long Dyn Inversion: alpha_dot ->q/Completed ==
  alpha_dot_c : Inport
  All_meas : Inport  Port=2
  A_w_z : Selector  InputPortWidth=3  Indices=3
  Add : Sum
  Bus Selector : BusSelector  OutputSignals=signal1.AoA meas (rad),signal1.omega_b meas (rad/s),signal1.SS meas (rad),signal1.V_TAS (m/s),signal2.A_w_CG
  Display : Display
  Display1 : Display
  Display2 : Display
  Divide{,1..3} (4 alike) : Product  Inputs=**
  Divide4 : Product  Inputs=/*
  Selector : Selector  InputPortWidth=3
  Selector1 : Selector  InputPortWidth=3  Indices=3
  Trigonometric Function : Trigonometry  Operator=sincos
  Trigonometric Function1 : Trigonometry  Operator=tan
  Trigonometric Function2 : Trigonometry  Operator=cos
  "q_c " : Sum  Inputs=++-
  q_c : Outport
  wires:
  Trigonometric Function/1 -> Divide1/1
  Bus Selector/1 -> Trigonometric Function/1  "<AoA meas (rad)>"
  Selector/1 -> Divide/2
  Bus Selector/2 -> Selector1/1, Selector/1  "<omega_b meas (rad/s)>"
  Divide2/1 -> "q_c "/2, Display1/1
  Selector1/1 -> Divide1/2
  Divide3/1 -> Divide4/1
  alpha_dot_c/1 -> "q_c "/1, Display/1
  All_meas/1 -> Bus Selector/1
  Bus Selector/5 -> A_w_z/1  "<A_w_CG>"
  Bus Selector/3 -> Trigonometric Function1/1, Trigonometric Function2/1  "<SS meas (rad)>"
  Divide4/1 -> "q_c "/3
  "q_c "/1 -> q_c/1
  Divide/1 -> Add/1
  Bus Selector/4 -> Divide3/2  "<V_TAS (m/s)>"
  Add/1 -> Divide2/1
  Trigonometric Function1/1 -> Divide2/2
  Divide1/1 -> Add/2
  Trigonometric Function2/1 -> Divide3/1
  Trigonometric Function/2 -> Divide/1
  A_w_z/1 -> Display2/1, Divide4/2

== system F16ASYM_Controlled/Primary Controller/P cont + adaptive Crossed NN + AWU+Lim ONELAYER/Long Dyn Inversion: alpha_dot ->q/Simplified ==
  alpha_dot_c : Inport
  All_meas : Inport  Port=2
  A_b_z : Selector  InputPortWidth=3  Indices=3
  Bus Selector : BusSelector  OutputSignals=signal2.A_b_CG,signal1.V_TAS (m/s)
  Display : Display
  Divide4 : Product  Inputs=*/
  "q_c " : Sum  Inputs=+-
  q_c : Outport
  wires:
  "q_c "/1 -> q_c/1
  All_meas/1 -> Bus Selector/1
  alpha_dot_c/1 -> "q_c "/1, Display/1
  Bus Selector/2 -> Divide4/2  "<V_TAS (m/s)>"
  Divide4/1 -> "q_c "/2
  A_b_z/1 -> Divide4/1  "A_b_z"
  Bus Selector/1 -> A_b_z/1  "<A_b_CG>"

== system F16ASYM_Controlled/Primary Controller/P cont + adaptive Crossed NN + AWU+Lim ONELAYER/Longitudinal Controller: AoA or A_w_z/Longitudinal controller in A_w_z ==
  A_w_z des : Inport
  AoA des (rad) : Inport  Port=2
  Anti-windup A_w_z : Inport  Port=3
  Anti-windup AoA : Inport  Port=4
  All meas : Inport  Port=5
  Accel rate --> AoA rate! : Subsystem
  Bus Creator : BusCreator  Inputs=5
  Bus Selector : BusSelector  OutputSignals=signal2.A_w_CG
  Divide : Product  Inputs=**
  Gain : Gain  Gain=-1
  Ground : Ground
  Ref Model and P Controller : Adaptive_FaultTolerantControl/Ref Model and P Controller  tau=2  y_i=0  K_f=1  K_b=1
  Selector : Selector  InputPortWidth=3  Indices=3
  Stall protection : Subsystem  Commented=on
  Sum : Sum  Inputs=+-|
  Terminator : Terminator
  Terminator1 : Terminator
  Terminator2 : Terminator
  A_chanel vars : Outport
  alpha_chanel vars : Outport  Port=2
  alpha_dot_c : Outport  Port=3
  wires:
  Anti-windup AoA/1 -> Terminator1/1
  AoA des (rad)/1 -> Terminator/1
  Selector/1 -> Gain/1
  Gain/1 -> Ref Model and P Controller/2
  Bus Selector/1 -> Selector/1  "<A_w_CG>"
  Anti-windup A_w_z/1 -> Terminator2/1
  A_w_z des/1 -> Ref Model and P Controller/1
  Ref Model and P Controller/1 -> Divide/1
  Ref Model and P Controller/2 -> Bus Creator/1  "A_sf_dot"
  Ref Model and P Controller/3 -> Bus Creator/2, Sum/1  "A_sf"
  Sum/1 -> Bus Creator/3  "A_err"
  Ref Model and P Controller/4 -> Sum/2
  Ref Model and P Controller/5 -> Bus Creator/4  "K_b_A"
  Bus Creator/1 -> A_chanel vars/1
  Ground/1 -> alpha_chanel vars/1
  Divide/1 -> alpha_dot_c/1
  Accel rate --> AoA rate!/1(A_w  to AoA rates factor) -> Bus Creator/5, Divide/2  "FactorF"
  All meas/1 -> Bus Selector/1, Stall protection/2(All meas), Accel rate --> AoA rate!/1(All_meas)

== system F16ASYM_Controlled/Primary Controller/P cont + adaptive Crossed NN + AWU+Lim ONELAYER/Longitudinal Controller: AoA or A_w_z/Longitudinal controller in AoA ==
  A_w_z des : Inport
  AoA des (rad) : Inport  Port=2
  Anti-windup A_w_z : Inport  Port=3
  Anti-windup AoA : Inport  Port=4
  All meas : Inport  Port=5
  Bus Creator : BusCreator
  Bus Selector : BusSelector  OutputSignals=signal1.AoA meas (rad)
  Ground : Ground
  Ref Model and P Controller : Adaptive_FaultTolerantControl/Ref Model and P Controller  tau=0.6  y_i=trim_state(8)  K_f=1  K_b=3.5
  Sum : Sum  Inputs=+-|
  Terminator : Terminator
  Terminator1 : Terminator
  Terminator2 : Terminator
  A_chanel vars : Outport
  alpha_chanel vars : Outport  Port=2
  alpha_dot_c : Outport  Port=3
  wires:
  All meas/1 -> Bus Selector/1
  Ref Model and P Controller/1 -> alpha_dot_c/1
  Bus Selector/1 -> Ref Model and P Controller/2  "<AoA meas (rad)>"
  AoA des (rad)/1 -> Ref Model and P Controller/1
  A_w_z des/1 -> Terminator/1
  Anti-windup A_w_z/1 -> Terminator1/1
  Anti-windup AoA/1 -> Terminator2/1
  Ref Model and P Controller/2 -> Bus Creator/1  "alpha_sf_dot"
  Ref Model and P Controller/3 -> Sum/1, Bus Creator/2  "alpha_sf"
  Sum/1 -> Bus Creator/3  "alpha_err"
  Bus Creator/1 -> alpha_chanel vars/1
  Ref Model and P Controller/4 -> Sum/2
  Ref Model and P Controller/5 -> Bus Creator/4  "K_b_alpha"
  Ground/1 -> A_chanel vars/1

== system F16ASYM_Controlled/Primary Controller/P cont + adaptive Crossed NN + AWU+Lim ONELAYER/Physical limitation/Moments ==
  C_L : Inport
  C_M : Inport  Port=2
  C_N : Inport  Port=3
  q : Inport  Port=4
  B span : Constant  Value=9.144
  CMA : Constant  Value=3.45
  Divide : Product  Inputs=**
  Divide1 : Product  Inputs=***
  Divide2 : Product  Inputs=**
  Divide3 : Product  Inputs=***
  Divide4 : Product  Inputs=**
  S_w : Constant  Value=27.87
  S_w1 : Constant  Value=27.87
  q1 : InportShadow  Port=4
  L : Outport
  M : Outport  Port=2
  N : Outport  Port=3
  wires:
  Divide4/1 -> M/1  "M"
  Divide3/1 -> Divide4/2
  C_M/1 -> Divide4/1
  CMA/1 -> Divide3/3
  S_w1/1 -> Divide3/2
  q1/1 -> Divide3/1
  Divide2/1 -> N/1  "N"
  C_N/1 -> Divide2/2
  Divide/1 -> L/1  "L"
  Divide1/1 -> Divide/2, Divide2/1
  C_L/1 -> Divide/1
  B span/1 -> Divide1/3
  S_w/1 -> Divide1/2
  q/1 -> Divide1/1

== system F16ASYM_Controlled/Primary Controller/P controller/Long Dyn Inversion: alpha_dot ->q/Completed ==
  alpha_dot_c : Inport
  All_meas : Inport  Port=2
  A_w_z : Selector  InputPortWidth=3  Indices=3
  Add : Sum
  Bus Selector : BusSelector  OutputSignals=signal1.AoA meas (rad),signal1.omega_b meas (rad/s),signal1.SS meas (rad),signal1.V_TAS (m/s),signal2.A_w_CG
  Display : Display
  Display1 : Display
  Display2 : Display
  Divide{,1..3} (4 alike) : Product  Inputs=**
  Divide4 : Product  Inputs=/*
  Selector : Selector  InputPortWidth=3
  Selector1 : Selector  InputPortWidth=3  Indices=3
  Trigonometric Function : Trigonometry  Operator=sincos
  Trigonometric Function1 : Trigonometry  Operator=tan
  Trigonometric Function2 : Trigonometry  Operator=cos
  "q_c " : Sum  Inputs=++-
  q_c : Outport
  wires:
  A_w_z/1 -> Divide4/2, Display2/1
  Trigonometric Function/2 -> Divide/1
  Trigonometric Function2/1 -> Divide3/1
  Divide1/1 -> Add/2
  Trigonometric Function1/1 -> Divide2/2
  Add/1 -> Divide2/1
  Bus Selector/4 -> Divide3/2  "<V_TAS (m/s)>"
  Divide/1 -> Add/1
  "q_c "/1 -> q_c/1
  Divide4/1 -> "q_c "/3
  Bus Selector/3 -> Trigonometric Function2/1, Trigonometric Function1/1  "<SS meas (rad)>"
  Bus Selector/5 -> A_w_z/1  "<A_w_CG>"
  All_meas/1 -> Bus Selector/1
  alpha_dot_c/1 -> Display/1, "q_c "/1
  Divide3/1 -> Divide4/1
  Selector1/1 -> Divide1/2
  Divide2/1 -> Display1/1, "q_c "/2
  Bus Selector/2 -> Selector/1, Selector1/1  "<omega_b meas (rad/s)>"
  Selector/1 -> Divide/2
  Bus Selector/1 -> Trigonometric Function/1  "<AoA meas (rad)>"
  Trigonometric Function/1 -> Divide1/1

== system F16ASYM_Controlled/Primary Controller/P controller/Long Dyn Inversion: alpha_dot ->q/Simplified ==
  alpha_dot_c : Inport
  All_meas : Inport  Port=2
  A_b_z : Selector  InputPortWidth=3  Indices=3
  Bus Selector : BusSelector  OutputSignals=signal2.A_b_CG,signal1.V_TAS (m/s)
  Display : Display
  Divide4 : Product  Inputs=*/
  "q_c " : Sum  Inputs=+-
  q_c : Outport
  wires:
  Bus Selector/1 -> A_b_z/1  "<A_b_CG>"
  A_b_z/1 -> Divide4/1  "A_b_z"
  Divide4/1 -> "q_c "/2
  Bus Selector/2 -> Divide4/2  "<V_TAS (m/s)>"
  alpha_dot_c/1 -> Display/1, "q_c "/1
  All_meas/1 -> Bus Selector/1
  "q_c "/1 -> q_c/1

== system F16ASYM_Controlled/Primary Controller/P controller/Longitudinal Controller: AoA or A_w_z/Longitudinal controller in A_w_z ==
  A_w_z des : Inport
  AoA des (rad) : Inport  Port=2
  Anti-windup A_w_z : Inport  Port=3
  Anti-windup AoA : Inport  Port=4
  All meas : Inport  Port=5
  Accel rate --> AoA rate! : Subsystem
  Bus Creator : BusCreator
  Bus Selector : BusSelector  OutputSignals=signal2.A_w_CG
  Gain : Gain  Gain=-1
  Ground : Ground
  Ref Model and P Controller : Adaptive_FaultTolerantControl/Ref Model and P Controller  tau=0.3  y_i=0  K_f=1  K_b=2
  Selector : Selector  InputPortWidth=3  Indices=3
  Sum : Sum  Inputs=+-|
  Terminator : Terminator
  Terminator1 : Terminator
  Terminator2 : Terminator
  A_chanel vars : Outport
  alpha_chanel vars : Outport  Port=2
  alpha_dot_c : Outport  Port=3
  wires:
  Ground/1 -> alpha_chanel vars/1
  Bus Creator/1 -> A_chanel vars/1
  Ref Model and P Controller/5 -> Bus Creator/4  "K_b_A"
  Ref Model and P Controller/4 -> Sum/2
  Sum/1 -> Bus Creator/3  "A_err"
  Ref Model and P Controller/3 -> Sum/1, Bus Creator/2  "A_sf"
  Ref Model and P Controller/2 -> Bus Creator/1  "A_sf_dot"
  Ref Model and P Controller/1 -> Accel rate --> AoA rate!/1(A_w_z dot)
  A_w_z des/1 -> Ref Model and P Controller/1
  Anti-windup A_w_z/1 -> Terminator2/1
  All meas/1 -> Accel rate --> AoA rate!/2(All_meas), Bus Selector/1
  Bus Selector/1 -> Selector/1  "<A_w_CG>"
  Accel rate --> AoA rate!/1(alpha_dot des) -> alpha_dot_c/1
  Gain/1 -> Ref Model and P Controller/2
  Selector/1 -> Gain/1
  AoA des (rad)/1 -> Terminator/1
  Anti-windup AoA/1 -> Terminator1/1

== system F16ASYM_Controlled/Primary Controller/P controller/Longitudinal Controller: AoA or A_w_z/Longitudinal controller in AoA ==
  A_w_z des : Inport
  AoA des (rad) : Inport  Port=2
  Anti-windup A_w_z : Inport  Port=3
  Anti-windup AoA : Inport  Port=4
  All meas : Inport  Port=5
  Bus Creator : BusCreator
  Bus Selector : BusSelector  OutputSignals=signal1.AoA meas (rad)
  Ground : Ground
  Ref Model and P Controller : Adaptive_FaultTolerantControl/Ref Model and P Controller  tau=0.8  y_i=trim_state(8)  K_f=1  K_b=2
  Sum : Sum  Inputs=+-|
  Terminator : Terminator
  Terminator1 : Terminator
  Terminator2 : Terminator
  A_chanel vars : Outport
  alpha_chanel vars : Outport  Port=2
  alpha_dot_c : Outport  Port=3
  wires:
  Ground/1 -> A_chanel vars/1
  Ref Model and P Controller/5 -> Bus Creator/4  "K_b_alpha"
  Ref Model and P Controller/4 -> Sum/2
  Bus Creator/1 -> alpha_chanel vars/1
  Sum/1 -> Bus Creator/3  "alpha_err"
  Ref Model and P Controller/3 -> Bus Creator/2, Sum/1  "alpha_sf"
  Ref Model and P Controller/2 -> Bus Creator/1  "alpha_sf_dot"
  Anti-windup AoA/1 -> Terminator2/1
  Anti-windup A_w_z/1 -> Terminator1/1
  A_w_z des/1 -> Terminator/1
  AoA des (rad)/1 -> Ref Model and P Controller/1
  Bus Selector/1 -> Ref Model and P Controller/2  "<AoA meas (rad)>"
  Ref Model and P Controller/1 -> alpha_dot_c/1
  All meas/1 -> Bus Selector/1

== system F16ASYM_Controlled/Primary Controller/P controller + adaptive Crossed NN/Complete crossed On-line (adaptive) multi-layer NN/Complete crossed On-line (adaptive) multi-layer NN: A_w_z ==
  v_ad^ prev : Inport
  All_meas : Inport  Port=2
  NN variables : Inport  Port=3
  B : Constant  Value=[1 0 0;0 0 0;0 1 0;0 0 0;0 0 1]
  Bus Selector : BusSelector  OutputSignals=p_chanel_vars,Long chanel,beta_r_chanel
  Bus Selector1 : BusSelector  OutputSignals=p_err,p_sf,p_sf_dot,K_b_p
  Bus Selector2 : BusSelector  OutputSignals=signal1.Alt meas (m),signal2.Mach,signal1.AoA meas (rad),signal1.SS meas (rad),signal1.omega_b meas (rad/s)
  Bus Selector4 : BusSelector  OutputSignals=beta_chanel vars.beta_err,r_chanel vars.r_err,beta_chanel vars.beta_sf,beta_chanel vars.beta_sf_dot,r_chanel vars.r_sf_dot,beta_chanel vars.K_b_beta,r_chanel vars.K_b_r
  Bus Selector5 : BusSelector  OutputSignals=A_chanel vars.A_err,q_chanel_vars.q_err,A_chanel vars.A_sf,A_chanel vars.A_sf_dot,q_chanel_vars.q_sf_dot,A_chanel vars.K_b_A,q_chanel_vars.K_b_q,A_chanel vars.FactorF
  C learning rate : Constant  Value=30  SampleTime=T_sim
  C reg param : Constant  SampleTime=T_sim
  Constant : Constant
  Cross NN A_w_z : MATLAB Function  TreatAsAtomicUnit=on
  Display : Display
  Divide : Product  Inputs=**
  Divide1 : Product  Inputs=**
  Memory2 : Memory  X0=V_Comp_A_w_z_last
  Memory3 : Memory  X0=W_Comp_A_w_z_last
  Mux1 : Mux  Inputs=9
  Mux10 : Mux  Inputs=3
  Mux{6..7,11..12} (4 alike) : Mux  Inputs=2
  Mux2 : Mux  Inputs=3
  Mux5 : Mux  Inputs=5
  Mux8 : Mux  Inputs=5
  Mux9 : Mux  Inputs=[9 3 5 5 3]
  Scope : Scope
      settings: SaveName=ScopeData8
  Selector : Selector  InputPortWidth=3
  Selector1 : Selector  InputPortWidth=3  Indices=3
  Terminator : Terminator
  Terminator1 : Terminator
  To Workspace : ToWorkspace  VariableName=V_Comp_A_w_z_last  SampleTime=-1
      settings: MaxDataPoints=1
  To Workspace1 : ToWorkspace  VariableName=W_Comp_A_w_z_last  SampleTime=-1
      settings: MaxDataPoints=1
  dem-less : Gain  Gain=T_sim
  dem-less3 : Gain  Gain=T_sim
  dem-less4 : Gain  Gain=T_sim^2
  dim-less : Gain  Gain=1/15000
  dim-less1 : Gain  Gain=T_sim
  dim-less2 : Gain  Gain=T_sim^2
  scaling1 : Gain  Gain=1/(9*9.81)
  scaling2 : Gain  Gain=1/(9*9.81)
  scaling3 : Gain  Gain=1/(9*9.81)
  v_ad^ : Outport
  wires:
  Bus Selector/3 -> Bus Selector4/1  "<beta_r_chanel>"
  Bus Selector/1 -> Bus Selector1/1  "<p_chanel_vars>"
  NN variables/1 -> Bus Selector/1
  Bus Selector2/5 -> Selector1/1, Selector/1  "<omega_b meas (rad/s)>"
  dim-less/1 -> Mux1/2
  Divide1/1 -> Mux1/6
  Divide/1 -> Mux1/4
  Bus Selector2/1 -> dim-less/1  "<Alt meas (m)>"
  All_meas/1 -> Bus Selector2/1
  Constant/1 -> Mux1/1
  Bus Selector1/3 -> dem-less/1  "<p_sf_dot>"
  Selector/1 -> Mux1/8
  Bus Selector2/4 -> Mux1/7  "<SS meas (rad)>"
  Bus Selector2/2 -> Divide/2, Mux1/3, Divide/1  "<Mach>"
  Bus Selector2/3 -> Divide1/1, Mux1/5, Divide1/2  "<AoA meas (rad)>"
  Bus Selector1/4 -> [K_roll]  "<K_b_p>"
  Bus Selector1/2 -> Mux2/2  "<p_sf>"
  Bus Selector1/1 -> [e_roll], Mux2/1  "<p_err>"
  dem-less/1 -> Mux2/3
  Mux12/1 -> [Ks_long]
  dem-less3/1 -> Mux8/4
  Bus Selector4/3 -> Mux8/3  "<beta_sf>"
  Bus Selector4/4 -> dem-less3/1  "<beta_sf_dot>"
  Bus Selector4/5 -> dem-less4/1  "<r_sf_dot>"
  Bus Selector4/7 -> Mux6/2  "<K_b_r>"
  Bus Selector4/6 -> Mux6/1  "<K_b_beta>"
  Mux6/1 -> [Ks_yaw]
  Bus Selector4/1 -> Mux8/1, Mux7/1  "<beta_err>"
  Bus Selector4/2 -> Mux8/2, Mux7/2  "<r_err>"
  Mux7/1 -> [e_yaw]  "e"
  dem-less4/1 -> Mux8/5
  Mux1/1 -> Mux9/1
  Mux2/1 -> Mux9/2
  Mux5/1 -> Mux9/3
  Mux8/1 -> Mux9/4
  v_ad^ prev/1 -> Mux9/5
  Mux9/1 -> Scope/1, Display/1, Cross NN A_w_z/1(X_bar)
  Cross NN A_w_z/3(Z_norm_unit) -> Terminator1/1
  C reg param/1 -> Cross NN A_w_z/9(Reg_param)
  C learning rate/1 -> Cross NN A_w_z/8(Learnign_rate)
  Cross NN A_w_z/1(v_ad_comp) -> v_ad^/1
  Memory2/1 -> Cross NN A_w_z/11(V)
  Memory3/1 -> Cross NN A_w_z/10(W)
  B/1 -> Cross NN A_w_z/7(B)
  Cross NN A_w_z/2(v_ad) -> Terminator/1
  Cross NN A_w_z/5(V_update) -> To Workspace/1, Memory2/1
  Cross NN A_w_z/4(W_update) -> Memory3/1, To Workspace1/1
  Mux10/1 -> Cross NN A_w_z/2(e)
  [e_roll] -> Mux10/1
  [e_long] -> Mux10/2
  [e_yaw] -> Mux10/3
  [K_roll] -> Cross NN A_w_z/4(K_roll)
  [Ks_long] -> Cross NN A_w_z/5(Ks_long)
  [Ks_yaw] -> Cross NN A_w_z/6(Ks_yaw)
  Selector1/1 -> Mux1/9
  dim-less1/1 -> scaling3/1
  scaling2/1 -> Mux5/1
  Bus Selector5/6 -> Mux12/1  "<K_b_A>"
  Bus Selector5/7 -> Mux12/2  "<K_b_q>"
  Bus Selector5/5 -> dim-less2/1  "<q_sf_dot>"
  Bus Selector5/4 -> dim-less1/1  "<A_sf_dot>"
  Bus Selector5/3 -> scaling1/1  "<A_sf>"
  Bus Selector5/2 -> Mux5/2, Mux11/2  "<q_err>"
  Bus Selector5/1 -> scaling2/1, Mux11/1  "<A_err>"
  Bus Selector/2 -> Bus Selector5/1  "<Long chanel>"
  Mux11/1 -> [e_long]  "e"
  scaling1/1 -> Mux5/3
  dim-less2/1 -> Mux5/5
  scaling3/1 -> Mux5/4
  Bus Selector5/8 -> [Factor_F]  "<FactorF>"
  [Factor_F] -> Cross NN A_w_z/3(Factor_F)
